simulink model "Scenario_MinimumExample_TwithoutTrafficLights_tol"  (R2021a)
settings: Solver=VariableStepAuto  StartTime=0.0  StopTime=50  RelTol=1e-3
model workspace (MAT data in the model file):
  Kz_dif = Simulink.Parameter
  Kz_dif.Value = Simulink.data.Expression
  Kz_dif.Value.ExpressionString = " L_dif / (Lc + ds)"
  Kz_dif.DataType = 'auto'
  Kz_dif.Dimensions = -1
  Kz_il = Simulink.Parameter
  Kz_il.Value = Simulink.data.Expression
  Kz_il.Value.ExpressionString = " L_il / (Lc + ds)"
  Kz_il.DataType = 'auto'
  Kz_il.Dimensions = -1
  Kz_ir = Simulink.Parameter
  Kz_ir.Value = Simulink.data.Expression
  Kz_ir.Value.ExpressionString = " L_ir / (Lc + ds)"
  Kz_ir.DataType = 'auto'
  Kz_ir.Dimensions = -1
  Kz_is = Simulink.Parameter
  Kz_is.Value = Simulink.data.Expression
  Kz_is.Value.ExpressionString = " L_is / (Lc + ds)"
  Kz_is.DataType = 'auto'
  Kz_is.Dimensions = -1
  Kz_long = Simulink.Parameter
  Kz_long.Value = Simulink.data.Expression
  Kz_long.Value.ExpressionString = " L_long / (Lc + ds)"
  Kz_long.Description = 'Segmentkapazität (wie viele autos passen hinein)'
  Kz_long.DataType = 'auto'
  Kz_long.Dimensions = -1
  Kz_pre = Simulink.Parameter
  Kz_pre.Value = Simulink.data.Expression
  Kz_pre.Value.ExpressionString = " L_pre / (Lc + ds)"
  Kz_pre.DataType = 'auto'
  Kz_pre.Dimensions = -1
  L_dif = Simulink.Parameter
  L_dif.Value = Simulink.data.Expression
  L_dif.Value.ExpressionString = "L_long-L_pre"
  L_dif.Description = 'Differenz zwischen Abbiegerspurlänge und normaler straßenlänge'
  L_dif.DataType = 'auto'
  L_dif.Dimensions = -1
  L_il = Simulink.Parameter
  L_il.Value = 30
  L_il.Description = 'Länge der innenkreuzungssegments, das linksabbieger durchqueren'
  L_il.DataType = 'auto'
  L_il.Dimensions = [1 1]
  L_ir = Simulink.Parameter
  L_ir.Value = 23
  L_ir.Description = 'Länge der innenkreuzungssegments, das rechtsabbieger durchqueren'
  L_ir.DataType = 'auto'
  L_ir.Dimensions = [1 1]
  L_is = Simulink.Parameter
  L_is.Value = 35
  L_is.Description = 'Länge der innenkreuzungssegments, das geradeausfahrer durchqueren'
  L_is.DataType = 'auto'
  L_is.Dimensions = [1 1]
  L_long = Simulink.Parameter
  L_long.Value = 52.8
  L_long.Description = 'Langes straßensegment  (52.8 meter)'
  L_long.DataType = 'auto'
  L_long.Dimensions = [1 1]
  L_pre = Simulink.Parameter
  L_pre.Value = 20
  L_pre.Description = 'Länge der Abbiegespuren'
  L_pre.DataType = 'auto'
  L_pre.Dimensions = [1 1]
  Lc = Simulink.Parameter
  Lc.Value = 4.4
  Lc.Description = 'Länge eines autos'
  Lc.DataType = 'auto'
  Lc.Dimensions = [1 1]
  Rk = Simulink.Parameter
  Rk.Value = Simulink.data.Expression
  Rk.Value.ExpressionString = " 1 / (Lc / v)"
  Rk.Description = 'Flussrate zwischen den Kanten (bei speed v)'
  Rk.DataType = 'auto'
  Rk.Dimensions = -1
  Tz_dif = Simulink.Parameter
  Tz_dif.Value = Simulink.data.Expression
  Tz_dif.Value.ExpressionString = " L_dif / v"
  Tz_dif.DataType = 'auto'
  Tz_dif.Dimensions = -1
  Tz_il = Simulink.Parameter
  Tz_il.Value = Simulink.data.Expression
  Tz_il.Value.ExpressionString = " L_il / v"
  Tz_il.DataType = 'auto'
  Tz_il.Dimensions = -1
  Tz_ir = Simulink.Parameter
  Tz_ir.Value = Simulink.data.Expression
  Tz_ir.Value.ExpressionString = " L_ir / v"
  Tz_ir.DataType = 'auto'
  Tz_ir.Dimensions = -1
  Tz_is = Simulink.Parameter
  Tz_is.Value = Simulink.data.Expression
  Tz_is.Value.ExpressionString = " L_is / v"
  Tz_is.DataType = 'auto'
  Tz_is.Dimensions = -1
  Tz_long = Simulink.Parameter
  Tz_long.Value = Simulink.data.Expression
  Tz_long.Value.ExpressionString = " L_long / v"
  Tz_long.Description = 'Segment durchfahrtzeit: wie lange würde ein auto brauchen,um
    | ungehindert durch das segment zu fahren.'
  Tz_long.DataType = 'auto'
  Tz_long.Dimensions = -1
  Tz_pre = Simulink.Parameter
  Tz_pre.Value = Simulink.data.Expression
  Tz_pre.Value.ExpressionString = " L_pre / v"
  Tz_pre.DataType = 'auto'
  Tz_pre.Dimensions = -1
  ds = Simulink.Parameter
  ds.Value = Simulink.data.Expression
  ds.Value.ExpressionString = "v*dt"
  ds.DataType = 'auto'
  ds.Dimensions = -1
  dt = Simulink.Parameter
  dt.Value = 1
  dt.Description = 'temporaler sicherheitsabstand'
  dt.DataType = 'auto'
  dt.Dimensions = [1 1]
  v = Simulink.Parameter
  v.Value = 13.89
  v.Description = 'geschwindigkeit eines autos
    | (km/h : 3.75 = m/s)
    | 	30km/h = 8,34m/s
    | 	20km/h = 5.56m/s
    | 	50km/h = 13.89m/s
    | '
  v.DataType = 'auto'
  v.Dimensions = [1 1]
libraries: StreetLanesLibrary x72, EdgesLibrary x64, MeasuringLibrary x34, SourcesAndSinksLibrary x11
(part 1 of 2)
settings Model: Creator=phill  LastModifiedBy=phill
settings SolverCC: ZeroCrossAlgorithm=Adaptive

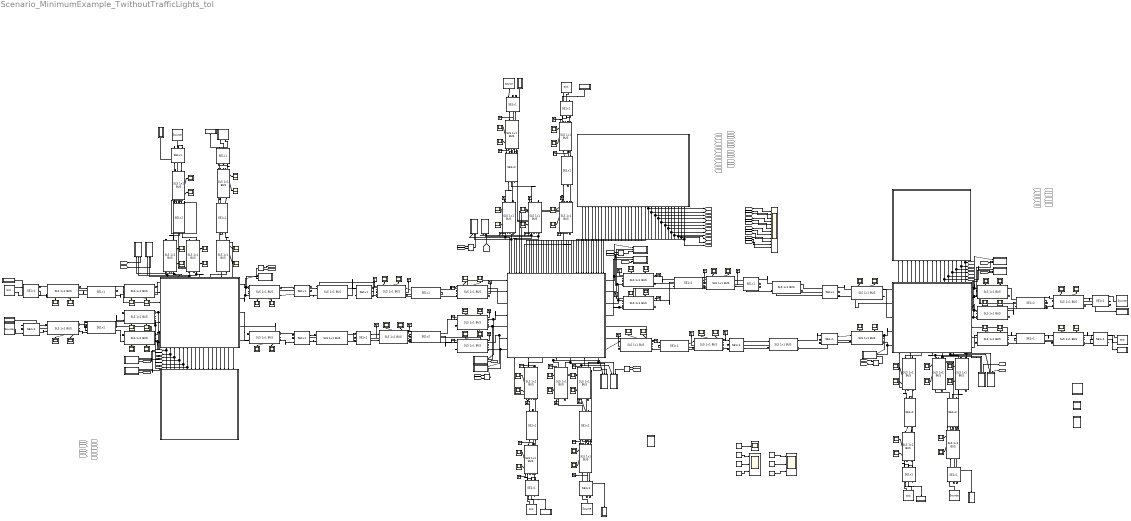
== system Scenario_MinimumExample_TwithoutTrafficLights_tol ==
  note: Controllers with tolerance
  Ain : StreetLanesLibrary/SLS 1x1 BUS  Kz=Kz_dif  Tz=Tz_dif
  Ain1 : StreetLanesLibrary/SLS 1x1 BUS  Kz=Kz_dif  Tz=Tz_dif
  Ain2 : StreetLanesLibrary/SLS 1x1 BUS  Kz=Kz_dif  Tz=Tz_dif
  AinSplit : EdgesLibrary/SE1x2  Rk1=0.5*Rk  Rk2=0.5*Rk
  AinSplit1 : EdgesLibrary/SE1x2  Rk1=0.5*Rk  Rk2=0.5*Rk
  AinSplit2 : EdgesLibrary/SE1x2  Rk1=0.5*Rk  Rk2=0.5*Rk
  AinX : Scope
  AinX1 : Scope
  AinX2 : Scope
  AinY : Scope
  AinY1 : Scope
  AinY2 : Scope
  Al : StreetLanesLibrary/SLS 1x1 BUS  Kz=Kz_pre  Tz=Tz_pre
  AlX : Scope
  AlY : Scope
  Ali : StreetLanesLibrary/SLS 1x1 BUS  Kz=Kz_pre  Tz=Tz_pre
  Ali1 : StreetLanesLibrary/SLS 1x1 BUS  Kz=Kz_pre  Tz=Tz_pre
  AliX : Scope
  AliX1 : Scope
  AliY : Scope
  AliY1 : Scope
  Ao : StreetLanesLibrary/SLS 1x1 BUS  Kz=Kz_pre  Tz=Tz_pre
  Ao1 : StreetLanesLibrary/SLS 1x1 BUS  Kz=Kz_pre  Tz=Tz_pre
  Ao2 : StreetLanesLibrary/SLS 1x1 BUS  Kz=Kz_pre  Tz=Tz_pre
  AoX : Scope
  AoX1 : Scope
  AoX2 : Scope
  AoY : Scope
  AoY1 : Scope
  AoY2 : Scope
  Aout : StreetLanesLibrary/SLS 1x1 BUS  Kz=Kz_dif  Tz=Tz_dif
  Aout1 : StreetLanesLibrary/SLS 1x1 BUS  Kz=Kz_dif  Tz=Tz_dif
  Aout2 : StreetLanesLibrary/SLS 1x1 BUS  Kz=Kz_dif  Tz=Tz_dif
  AoutX : Scope
  AoutX1 : Scope
  AoutX2 : Scope
  AoutY : Scope
  AoutY1 : Scope
  AoutY2 : Scope
  Ari : StreetLanesLibrary/SLS 1x1 BUS  Kz=Kz_pre  Tz=Tz_pre
  Ari1 : StreetLanesLibrary/SLS 1x1 BUS  Kz=Kz_pre  Tz=Tz_pre
  AriX : Scope
  AriX1 : Scope
  AriY : Scope
  AriY1 : Scope
  Ars : StreetLanesLibrary/SLS 1x1 BUS  Kz=Kz_pre  Tz=Tz_pre
  ArsX : Scope
  ArsY : Scope
  Bin : StreetLanesLibrary/SLS 1x1 BUS  Kz=Kz_dif  Tz=Tz_dif
  BinSplit1 : EdgesLibrary/SE1x2  Rk1=0.5*Rk  Rk2=0.5*Rk
  BinX : Scope
  BinY : Scope
  Bl : StreetLanesLibrary/SLS 1x1 BUS  Kz=Kz_pre  Tz=Tz_pre
  BlX : Scope
  BlY : Scope
  Bo : StreetLanesLibrary/SLS 1x1 BUS  Kz=Kz_pre  Tz=Tz_pre
  Bo1 : StreetLanesLibrary/SLS 1x1 BUS  Kz=Kz_pre  Tz=Tz_pre
  Bo2 : StreetLanesLibrary/SLS 1x1 BUS  Kz=Kz_pre  Tz=Tz_pre
  Bo3 : StreetLanesLibrary/SLS 1x1 BUS  Kz=Kz_long  Tz=Tz_long
  BoX : Scope
  BoX1 : Scope
  BoX2 : Scope
  BoY : Scope
  BoY1 : Scope
  BoY2 : Scope
  Bout : StreetLanesLibrary/SLS 1x1 BUS  Kz=Kz_dif  Tz=Tz_dif
  BoutX : Scope
  BoutY : Scope
  Brs : StreetLanesLibrary/SLS 1x1 BUS  Kz=Kz_pre  Tz=Tz_pre
  Brs1 : StreetLanesLibrary/SLS 1x1 BUS  Kz=Kz_pre  Tz=Tz_pre
  Brs2 : StreetLanesLibrary/SLS 1x1 BUS  Kz=Kz_pre  Tz=Tz_pre
  Brs3 : StreetLanesLibrary/SLS 1x1 BUS  Kz=Kz_long  Tz=Tz_long
  BrsX : Scope
  BrsX1 : Scope
  BrsX2 : Scope
  BrsY : Scope
  BrsY1 : Scope
  BrsY2 : Scope
  Chart1 : Stateflow chart  TreatAsAtomicUnit=on  mask{tol=0}
      mask prompts: tol "tolerance"
      settings: PortSchema="{\"entries\":[{\"content\":{\"sides\":[{\"content\":{\"connectorIds\":[]},\"type\":\"ConnectorPlacement.EquallySpacedRectSide\",\"uuid\":\"dee1a780-e9dd-4205-adb9-3e9cb1ec0cd6\"},{\"content\":{\"connectorIds\":[],\"side\":\"RIGHT\"},\"type\":\"ConnectorPlacement.EquallySpacedRectSide\",\"uuid\":\"bc6af08d-2df8-4a74-93d0-032b7c1c381c\"},{\"content\":{\"connectorIds\":[],\"side\":\"TOP\"},\"type\":\"ConnectorPlacement.EquallySpacedRectSide\",\"uuid\":\"98fea325-c9fc-472d-8e1a-d846d6e99e12\"},{\"content\":{\"connectorIds\":[\"In5\",\"In1\",\"In2\",\"In3\",\"In4\",\"In11\",\"In10\",\"In9\",\"In8\",\"In7\",\"In6\",\"Out5\",\"Out6\",\"Out1\",\"Out2\",\"Out3\",\"Out4\"],\"side\":\"BOTTOM\"},\"type\":\"ConnectorPlacement.EquallySpacedRectSide\",\"uuid\":\"a092283f-ef46-48e2-a5f8-8210ac00b2f9\"}]},\"type\":\"ConnectorPlacement.EquallySpacedConnector\",\"uuid\":\"33a851aa-4180-41c0-b4bb-9b9c3be41936\"}],\"packageUris\":[\"http://schema.mathworks.com/mf0/Connector/R2020b\"],\"version\":\"1.0\"}"
  Chart2 : Stateflow chart  TreatAsAtomicUnit=on  mask{tol=0}
      mask prompts: tol "tolerance"
      settings: PortSchema="{\"entries\":[{\"content\":{\"sides\":[{\"content\":{\"connectorIds\":[]},\"type\":\"ConnectorPlacement.EquallySpacedRectSide\",\"uuid\":\"dee1a780-e9dd-4205-adb9-3e9cb1ec0cd6\"},{\"content\":{\"connectorIds\":[],\"side\":\"RIGHT\"},\"type\":\"ConnectorPlacement.EquallySpacedRectSide\",\"uuid\":\"bc6af08d-2df8-4a74-93d0-032b7c1c381c\"},{\"content\":{\"connectorIds\":[],\"side\":\"TOP\"},\"type\":\"ConnectorPlacement.EquallySpacedRectSide\",\"uuid\":\"98fea325-c9fc-472d-8e1a-d846d6e99e12\"},{\"content\":{\"connectorIds\":[\"In5\",\"In1\",\"In2\",\"In3\",\"In4\",\"In11\",\"In10\",\"In9\",\"In8\",\"In7\",\"In6\",\"Out5\",\"Out6\",\"Out1\",\"Out2\",\"Out3\",\"Out4\"],\"side\":\"BOTTOM\"},\"type\":\"ConnectorPlacement.EquallySpacedRectSide\",\"uuid\":\"a092283f-ef46-48e2-a5f8-8210ac00b2f9\"}]},\"type\":\"ConnectorPlacement.EquallySpacedConnector\",\"uuid\":\"33a851aa-4180-41c0-b4bb-9b9c3be41936\"}],\"packageUris\":[\"http://schema.mathworks.com/mf0/Connector/R2020b\"],\"version\":\"1.0\"}"
  Cin : StreetLanesLibrary/SLS 1x1 BUS  Kz=Kz_dif  Tz=Tz_dif
  Cin1 : StreetLanesLibrary/SLS 1x1 BUS  Kz=Kz_dif  Tz=Tz_dif
  Cin2 : StreetLanesLibrary/SLS 1x1 BUS  Kz=Kz_dif  Tz=Tz_dif
  Cin3 : StreetLanesLibrary/SLS 1x1 BUS  Kz=Kz_long  Tz=Tz_long
  CinSplit : EdgesLibrary/SE1x2  Rk1=0.5*Rk  Rk2=0.5*Rk
  CinSplit1 : EdgesLibrary/SE1x2  Rk1=0.5*Rk  Rk2=0.5*Rk
  CinSplit2 : EdgesLibrary/SE1x2  Rk1=0.5*Rk  Rk2=0.5*Rk
  CinX : Scope
  CinX1 : Scope
  CinX2 : Scope
  CinY : Scope
  CinY1 : Scope
  CinY2 : Scope
  Cl : StreetLanesLibrary/SLS 1x1 BUS  Kz=Kz_pre  Tz=Tz_pre
  Cl1 : StreetLanesLibrary/SLS 1x1 BUS  Kz=Kz_pre  Tz=Tz_pre
  Cl2 : StreetLanesLibrary/SLS 1x1 BUS  Kz=Kz_pre  Tz=Tz_pre
  ClX : Scope
  ClX1 : Scope
  ClX2 : Scope
  ClY : Scope
  ClY1 : Scope
  Cly : Scope
  Co : StreetLanesLibrary/SLS 1x1 BUS  Kz=Kz_pre  Tz=Tz_pre
  Co1 : StreetLanesLibrary/SLS 1x1 BUS  Kz=Kz_pre  Tz=Tz_pre
  Co2 : StreetLanesLibrary/SLS 1x1 BUS  Kz=Kz_pre  Tz=Tz_pre
  CoX : Scope
  CoX1 : Scope
  CoX2 : Scope
  CoY : Scope
  CoY1 : Scope
  CoY2 : Scope
  Cout{,1..3} (4 alike) : StreetLanesLibrary/SLS 1x1 BUS  Kz=Kz_dif  Tz=Tz_dif
  CoutX : Scope
  CoutX1 : Scope
  CoutX2 : Scope
  CoutY : Scope
  CoutY1 : Scope
  CoutY2 : Scope
  Crs : StreetLanesLibrary/SLS 1x1 BUS  Kz=Kz_pre  Tz=Tz_pre
  CrsX : Scope
  CrsY : Scope
  Cs : StreetLanesLibrary/SLS 1x1 BUS  Kz=Kz_pre  Tz=Tz_pre
  Cs1 : StreetLanesLibrary/SLS 1x1 BUS  Kz=Kz_pre  Tz=Tz_pre
  CsX : Scope
  CsX1 : Scope
  CsY : Scope
  CsY1 : Scope
  Din : StreetLanesLibrary/SLS 1x1 BUS  Kz=Kz_dif  Tz=Tz_dif
  DinSplit : EdgesLibrary/SE1x2  Rk1=0.5*Rk  Rk2=0.5*Rk
  DinX : Scope
  DinY : Scope
  Dl : StreetLanesLibrary/SLS 1x1 BUS  Kz=Kz_pre  Tz=Tz_pre
  DlX : Scope
  DlY : Scope
  Do : StreetLanesLibrary/SLS 1x1 BUS  Kz=Kz_pre  Tz=Tz_pre
  DoX : Scope
  DoY : Scope
  Dout : StreetLanesLibrary/SLS 1x1 BUS  Kz=Kz_dif  Tz=Tz_dif
  DoutX : Scope
  DoutY : Scope
  Drs : StreetLanesLibrary/SLS 1x1 BUS  Kz=Kz_pre  Tz=Tz_pre
  DrsX : Scope
  DrsY : Scope
  From14 : From  Commented=on  GotoTag=LenCs
  From15 : From  Commented=on  GotoTag=LenCl
  From20 : From  Commented=on  GotoTag=LenAr
  From21 : From  Commented=on  GotoTag=LenAl
  From22 : From  Commented=on  GotoTag=LenBr
  From23 : From  Commented=on  GotoTag=LenBs
  From24 : From  Commented=on  GotoTag=CenAl
  From25 : From  Commented=on  GotoTag=CenAs
  From26 : From  Commented=on  GotoTag=CenDs
  From27 : From  Commented=on  GotoTag=CenDr
  From28 : From  Commented=on  GotoTag=CenAr
  From29 : From  Commented=on  GotoTag=CenBl
  From30 : From  Commented=on  GotoTag=CenBs
  From31 : From  Commented=on  GotoTag=CenBr
  From32 : From  Commented=on  GotoTag=CenCl
  From33 : From  Commented=on  GotoTag=CenCs
  From34 : From  Commented=on  GotoTag=CenCr
  From35 : From  Commented=on  GotoTag=CenDl
  From42 : From  Commented=on  GotoTag=RenCs
  From43 : From  Commented=on  GotoTag=RenCl
  From44 : From  Commented=on  GotoTag=RenAr
  From45 : From  Commented=on  GotoTag=RenAl
  From46 : From  Commented=on  GotoTag=RenBr
  From47 : From  Commented=on  GotoTag=RenBs
  Goto12 : Goto  Commented=on  GotoTag=LenCl
  Goto13 : Goto  Commented=on  GotoTag=LenCs
  Goto16 : Goto  Commented=on  GotoTag=LenBs
  Goto17 : Goto  Commented=on  GotoTag=LenBr
  Goto18 : Goto  Commented=on  GotoTag=LenAl
  Goto19 : Goto  Commented=on  GotoTag=LenAr
  Goto24 : Goto  Commented=on  GotoTag=CenAl
  Goto25 : Goto  Commented=on  GotoTag=CenAs
  Goto26 : Goto  Commented=on  GotoTag=CenDs
  Goto27 : Goto  Commented=on  GotoTag=CenDr
  Goto28 : Goto  Commented=on  GotoTag=CenAr
  Goto29 : Goto  Commented=on  GotoTag=CenBl
  Goto30 : Goto  Commented=on  GotoTag=CenBs
  Goto31 : Goto  Commented=on  GotoTag=CenBr
  Goto32 : Goto  Commented=on  GotoTag=CenCl
  Goto33 : Goto  Commented=on  GotoTag=CenCs
  Goto34 : Goto  Commented=on  GotoTag=CenCr
  Goto35 : Goto  Commented=on  GotoTag=CenDl
  Goto42 : Goto  Commented=on  GotoTag=RenCl
  Goto43 : Goto  Commented=on  GotoTag=RenCs
  Goto44 : Goto  Commented=on  GotoTag=RenBs
  Goto45 : Goto  Commented=on  GotoTag=RenBr
  Goto46 : Goto  Commented=on  GotoTag=RenAl
  Goto47 : Goto  Commented=on  GotoTag=RenAr
  Kz_dif : Constant  Value=Kz_dif
  Kz_long : Constant  Value=Kz_long
  Kz_pre : Constant  Value=Kz_pre
  Kzs : Scope  NumInputPorts=3
  Logical Operator{,1..5} (6 alike) : Logic  Operator=OR  AllPortsSameDT=off  OutDataTypeStr=boolean
  Plus-Controller : Stateflow chart  TreatAsAtomicUnit=on  mask{green_duration_sr=6, green_duration_l=6, tol=0}
      mask prompts: green_duration_sr "Green Duration for straight/right traffic"; green_duration_l "Green Duration for left traffic"; tol "tolerance"
      settings: PortSchema="{\"entries\":[{\"content\":{\"sides\":[{\"content\":{\"connectorIds\":[]},\"type\":\"ConnectorPlacement.EquallySpacedRectSide\",\"uuid\":\"2590cc03-86a2-4387-8b1b-fdf4c8b68aa6\"},{\"content\":{\"connectorIds\":[],\"side\":\"RIGHT\"},\"type\":\"ConnectorPlacement.EquallySpacedRectSide\",\"uuid\":\"b97063cd-dd31-425f-b4aa-3aaa013ac411\"},{\"content\":{\"connectorIds\":[],\"side\":\"TOP\"},\"type\":\"ConnectorPlacement.EquallySpacedRectSide\",\"uuid\":\"ef5846b9-436e-4b10-a854-1305521b6a0d\"},{\"content\":{\"connectorIds\":[\"In3\",\"In4\",\"In1\",\"In2\",\"In5\",\"In6\",\"In7\",\"In8\",\"In9\",\"In10\",\"In11\",\"In12\",\"In13\",\"In14\",\"In15\",\"In16\",\"In17\",\"In18\",\"In19\",\"In20\",\"Out1\",\"Out2\",\"Out3\",\"Out4\",\"Out5\",\"Out6\",\"Out7\",\"Out8\",\"Out9\",\"Out10\",\"Out11\",\"Out12\"],\"side\":\"BOTTOM\"},\"type\":\"ConnectorPlacement.EquallySpacedRectSide\",\"uuid\":\"44b73820-3b7c-4ee5-b5da-9465e85a924e\"}]},\"type\":\"ConnectorPlacement.EquallySpacedConnector\",\"uuid\":\"3342797d-7762-4a2a-891a-654024402a66\"}],\"packageUris\":[\"http://schema.mathworks.com/mf0/Connector/R2020b\"],\"version\":\"1.0\"}"
  Rk : Constant  Value=Rk
  SE1x{1..8} (8 alike) : EdgesLibrary/SE1x1  Rk=Rk  slope=2000
  Scope : Scope  NumInputPorts=12
  Sink A : SourcesAndSinksLibrary/Sink  SystemSampleTime=-1  VariantActivationTime=update diagram  Latency=0  AutoFrameSizeCalculation=off
      settings: PortSchema="{\"entries\":[{\"content\":{\"sides\":[{\"content\":{\"connectorIds\":[\"Out1\",\"Out2\"]},\"type\":\"ConnectorPlacement.EquallySpacedRectSide\",\"uuid\":\"9fd2383e-3590-4f0f-bafc-5a4adfbb32b4\"},{\"content\":{\"connectorIds\":[],\"side\":\"RIGHT\"},\"type\":\"ConnectorPlacement.EquallySpacedRectSide\",\"uuid\":\"1e687aa9-1098-45bd-a1f6-ea403f3f2897\"},{\"content\":{\"connectorIds\":[],\"side\":\"TOP\"},\"type\":\"ConnectorPlacement.EquallySpacedRectSide\",\"uuid\":\"fe6eaa71-085c-414b-983a-a0e72e52a49c\"}]},\"type\":\"ConnectorPlacement.EquallySpacedConnector\",\"uuid\":\"370c1712-4373-4726-99c2-6cb04807ece1\"}],\"packageUris\":[\"http://schema.mathworks.com/mf0/Connector/R2020b\"],\"version\":\"1.0\"}"
  Sink A1 : SourcesAndSinksLibrary/Sink  SystemSampleTime=-1  VariantActivationTime=update diagram  Latency=0  AutoFrameSizeCalculation=off
      settings: PortSchema="{\"entries\":[{\"content\":{\"sides\":[{\"content\":{\"connectorIds\":[\"Out1\",\"Out2\"]},\"type\":\"ConnectorPlacement.EquallySpacedRectSide\",\"uuid\":\"9fd2383e-3590-4f0f-bafc-5a4adfbb32b4\"},{\"content\":{\"connectorIds\":[],\"side\":\"RIGHT\"},\"type\":\"ConnectorPlacement.EquallySpacedRectSide\",\"uuid\":\"1e687aa9-1098-45bd-a1f6-ea403f3f2897\"},{\"content\":{\"connectorIds\":[],\"side\":\"TOP\"},\"type\":\"ConnectorPlacement.EquallySpacedRectSide\",\"uuid\":\"fe6eaa71-085c-414b-983a-a0e72e52a49c\"}]},\"type\":\"ConnectorPlacement.EquallySpacedConnector\",\"uuid\":\"370c1712-4373-4726-99c2-6cb04807ece1\"}],\"packageUris\":[\"http://schema.mathworks.com/mf0/Connector/R2020b\"],\"version\":\"1.0\"}"
  Sink A2 : Subsystem  AncestorBlock=SourcesAndSinksLibrary/Sink
      settings: PortSchema="{\"entries\":[{\"content\":{\"sides\":[{\"content\":{\"connectorIds\":[\"Out1\",\"Out2\"]},\"type\":\"ConnectorPlacement.EquallySpacedRectSide\",\"uuid\":\"9fd2383e-3590-4f0f-bafc-5a4adfbb32b4\"},{\"content\":{\"connectorIds\":[],\"side\":\"RIGHT\"},\"type\":\"ConnectorPlacement.EquallySpacedRectSide\",\"uuid\":\"1e687aa9-1098-45bd-a1f6-ea403f3f2897\"},{\"content\":{\"connectorIds\":[],\"side\":\"TOP\"},\"type\":\"ConnectorPlacement.EquallySpacedRectSide\",\"uuid\":\"fe6eaa71-085c-414b-983a-a0e72e52a49c\"}]},\"type\":\"ConnectorPlacement.EquallySpacedConnector\",\"uuid\":\"370c1712-4373-4726-99c2-6cb04807ece1\"}],\"packageUris\":[\"http://schema.mathworks.com/mf0/Connector/R2020b\"],\"version\":\"1.0\"}"
      mask Display: image('$imagefile'); % Use "Edit Image" on toolstrip to change.
  Sink C1 : SourcesAndSinksLibrary/Sink  SystemSampleTime=-1  VariantActivationTime=update diagram  Latency=0  AutoFrameSizeCalculation=off
      settings: PortSchema="{\"entries\":[{\"content\":{\"sides\":[{\"content\":{\"connectorIds\":[\"Out1\",\"Out2\"]},\"type\":\"ConnectorPlacement.EquallySpacedRectSide\",\"uuid\":\"9fd2383e-3590-4f0f-bafc-5a4adfbb32b4\"},{\"content\":{\"connectorIds\":[],\"side\":\"RIGHT\"},\"type\":\"ConnectorPlacement.EquallySpacedRectSide\",\"uuid\":\"1e687aa9-1098-45bd-a1f6-ea403f3f2897\"},{\"content\":{\"connectorIds\":[],\"side\":\"TOP\"},\"type\":\"ConnectorPlacement.EquallySpacedRectSide\",\"uuid\":\"fe6eaa71-085c-414b-983a-a0e72e52a49c\"}]},\"type\":\"ConnectorPlacement.EquallySpacedConnector\",\"uuid\":\"370c1712-4373-4726-99c2-6cb04807ece1\"}],\"packageUris\":[\"http://schema.mathworks.com/mf0/Connector/R2020b\"],\"version\":\"1.0\"}"
  Sink C2 : SourcesAndSinksLibrary/Sink  SystemSampleTime=-1  VariantActivationTime=update diagram  Latency=0  AutoFrameSizeCalculation=off
      settings: PortSchema="{\"entries\":[{\"content\":{\"sides\":[{\"content\":{\"connectorIds\":[\"Out1\",\"Out2\"]},\"type\":\"ConnectorPlacement.EquallySpacedRectSide\",\"uuid\":\"9fd2383e-3590-4f0f-bafc-5a4adfbb32b4\"},{\"content\":{\"connectorIds\":[],\"side\":\"RIGHT\"},\"type\":\"ConnectorPlacement.EquallySpacedRectSide\",\"uuid\":\"1e687aa9-1098-45bd-a1f6-ea403f3f2897\"},{\"content\":{\"connectorIds\":[],\"side\":\"TOP\"},\"type\":\"ConnectorPlacement.EquallySpacedRectSide\",\"uuid\":\"fe6eaa71-085c-414b-983a-a0e72e52a49c\"}]},\"type\":\"ConnectorPlacement.EquallySpacedConnector\",\"uuid\":\"370c1712-4373-4726-99c2-6cb04807ece1\"}],\"packageUris\":[\"http://schema.mathworks.com/mf0/Connector/R2020b\"],\"version\":\"1.0\"}"
  Sink D : SourcesAndSinksLibrary/Sink  SystemSampleTime=-1  VariantActivationTime=update diagram  Latency=0  AutoFrameSizeCalculation=off
      settings: PortSchema="{\"entries\":[{\"content\":{\"sides\":[{\"content\":{\"connectorIds\":[\"Out1\",\"Out2\"]},\"type\":\"ConnectorPlacement.EquallySpacedRectSide\",\"uuid\":\"9fd2383e-3590-4f0f-bafc-5a4adfbb32b4\"},{\"content\":{\"connectorIds\":[],\"side\":\"RIGHT\"},\"type\":\"ConnectorPlacement.EquallySpacedRectSide\",\"uuid\":\"1e687aa9-1098-45bd-a1f6-ea403f3f2897\"},{\"content\":{\"connectorIds\":[],\"side\":\"TOP\"},\"type\":\"ConnectorPlacement.EquallySpacedRectSide\",\"uuid\":\"fe6eaa71-085c-414b-983a-a0e72e52a49c\"}]},\"type\":\"ConnectorPlacement.EquallySpacedConnector\",\"uuid\":\"370c1712-4373-4726-99c2-6cb04807ece1\"}],\"packageUris\":[\"http://schema.mathworks.com/mf0/Connector/R2020b\"],\"version\":\"1.0\"}"
  Source A : SourcesAndSinksLibrary/Source  SystemSampleTime=-1  VariantActivationTime=update diagram  Latency=0  AutoFrameSizeCalculation=off
  Source A1 : SourcesAndSinksLibrary/Source  SystemSampleTime=-1  VariantActivationTime=update diagram  Latency=0  AutoFrameSizeCalculation=off
  Source A2 : SourcesAndSinksLibrary/Source  SystemSampleTime=-1  VariantActivationTime=update diagram  Latency=0  AutoFrameSizeCalculation=off
  Source C1 : SourcesAndSinksLibrary/Source  SystemSampleTime=-1  VariantActivationTime=update diagram  Latency=0  AutoFrameSizeCalculation=off
  Source C2 : SourcesAndSinksLibrary/Source  SystemSampleTime=-1  VariantActivationTime=update diagram  Latency=0  AutoFrameSizeCalculation=off
  Source D : SourcesAndSinksLibrary/Source  SystemSampleTime=-1  VariantActivationTime=update diagram  Latency=0  AutoFrameSizeCalculation=off
  Subsystem : Subsystem  mask{Kz_left=Kz_il, Tz_left=Tz_il, Kz_straight=Kz_is, Tz_straight=Tz_is, Kz_right=Kz_ir, Tz_right=Tz_ir, Rk=Rk}
      settings: PortSchema="{\"entries\":[{\"content\":{\"sides\":[{\"content\":{\"connectorIds\":[\"In1\",\"In2\",\"Out30\",\"In3\",\"Out31\",\"In4\",\"Out32\"]},\"type\":\"ConnectorPlacement.EquallySpacedRectSide\",\"uuid\":\"223afcc5-5490-41e2-b2c1-0ac31bdd31f0\"},{\"content\":{\"connectorIds\":[\"In25\",\"Out1\",\"In26\",\"Out2\",\"In27\",\"In28\",\"Out3\"],\"side\":\"RIGHT\"},\"type\":\"ConnectorPlacement.EquallySpacedRectSide\",\"uuid\":\"e803e5ea-345a-49fc-8782-ffb100729ba0\"},{\"content\":{\"connectorIds\":[\"In5\",\"Out7\",\"Out8\",\"In6\",\"In7\",\"In8\",\"Out9\",\"Out10\",\"Out11\",\"Out12\",\"Out13\",\"Out14\",\"Out15\",\"Out16\",\"Out17\",\"Out18\",\"Out19\",\"Out20\",\"Out21\",\"Out22\",\"Out23\",\"Out24\",\"Out25\",\"Out26\",\"Out27\",\"Out28\",\"Out29\",\"In9\",\"In10\",\"In11\",\"In12\",\"In13\",\"In14\",\"In15\",\"In16\",\"In17\",\"In18\",\"In19\",\"In20\"],\"side\":\"TOP\"},\"type\":\"ConnectorPlacement.EquallySpacedRectSide\",\"uuid\":\"8581fbf9-6742-4a7a-9e93-ed29b1a56c31\"},{\"content\":{\"connectorIds\":[\"In21\",\"In22\",\"Out4\",\"In23\",\"Out5\",\"In24\",\"Out6\"],\"side\":\"BOTTOM\"},\"type\":\"ConnectorPlacement.EquallySpacedRectSide\",\"uuid\":\"cc67de78-9dd9-463d-9445-caa2eb7c099b\"}]},\"type\":\"ConnectorPlacement.EquallySpacedConnector\",\"uuid\":\"ac6fc4cc-2326-4bcf-896c-a5d089a8f47a\"}],\"packageUris\":[\"http://schema.mathworks.com/mf0/Connector/R2020b\"],\"version\":\"1.0\"}"
      mask Display:
      | %image('$imagefile'); % Use "Edit Image" on toolstrip to change.
      | disp('+ \n\n');
      | KzS = get_param(gcb,'Kz_straight');
      | TzS = get_param(gcb,'Tz_straight');
      | KzR = get_param(gcb,'Kz_right');
      | TzR = get_param(gcb,'Tz_right');
      | KzL = get_param(gcb,'Kz_left');
      | TzL = get_param(gcb,'Tz_left');
      | Rk = get_param(gcb,'Rk');
      | disp(['Rk = ', Rk, ' | Kz/Tz L = ', KzL, ' ', TzL, ' | Kz/Tz S = ', KzS, ' ', TzS, ' | Kz/Tz R = ', KzR, ' ', TzR]);
  Subsystem1 : Subsystem  mask{Kz_left=Kz_il, Tz_left=Tz_il, Kz_straight=Kz_is, Tz_straight=Tz_is, Kz_right=Kz_ir, Tz_right=Tz_ir, Rk=Rk}
      settings: PortSchema="{\"entries\":[{\"content\":{\"sides\":[{\"content\":{\"connectorIds\":[\"In1\",\"In2\",\"Out18\",\"In3\",\"Out19\"]},\"type\":\"ConnectorPlacement.EquallySpacedRectSide\",\"uuid\":\"96c9f498-b0bc-4839-a476-8992d885d35a\"},{\"content\":{\"connectorIds\":[\"In14\",\"Out1\",\"In15\",\"Out2\",\"In16\",\"In17\",\"Out3\"],\"side\":\"RIGHT\"},\"type\":\"ConnectorPlacement.EquallySpacedRectSide\",\"uuid\":\"11ab0cdd-7db6-4f39-a252-8216aa6322d2\"},{\"content\":{\"connectorIds\":[\"Out7\",\"Out8\",\"Out9\",\"Out10\",\"Out11\",\"Out12\",\"Out13\",\"Out14\",\"Out15\",\"Out16\",\"Out17\",\"In4\",\"In5\",\"In6\",\"In7\",\"In8\",\"In9\"],\"side\":\"TOP\"},\"type\":\"ConnectorPlacement.EquallySpacedRectSide\",\"uuid\":\"f8ff7b80-df82-4633-b83a-80e44c4409b9\"},{\"content\":{\"connectorIds\":[\"In10\",\"In11\",\"Out4\",\"In12\",\"Out5\",\"In13\",\"Out6\"],\"side\":\"BOTTOM\"},\"type\":\"ConnectorPlacement.EquallySpacedRectSide\",\"uuid\":\"816219a6-152c-447e-807e-ad4d62c96b47\"}]},\"type\":\"ConnectorPlacement.EquallySpacedConnector\",\"uuid\":\"16c591aa-9a6b-4cb9-9c60-a78ca06e8a6b\"}],\"packageUris\":[\"http://schema.mathworks.com/mf0/Connector/R2020b\"],\"version\":\"1.0\"}"
      mask Display:
      | %image('$imagefile'); % Use "Edit Image" on toolstrip to change.
      | disp('T \n\n');
      | KzS = get_param(gcb,'Kz_straight');
      | TzS = get_param(gcb,'Tz_straight');
      | KzR = get_param(gcb,'Kz_right');
      | TzR = get_param(gcb,'Tz_right');
      | KzL = get_param(gcb,'Kz_left');
      | TzL = get_param(gcb,'Tz_left');
      | Rk = get_param(gcb,'Rk');
      | disp(['Rk = ', Rk, ' | Kz/Tz L = ', KzL, ' ', TzL, ' | Kz/Tz S = ', KzS, ' ', TzS, ' | Kz/Tz R = ', KzR, ' ', TzR]);
  Subsystem2 : Subsystem  mask{Kz_left=Kz_il, Tz_left=Tz_il, Kz_straight=Kz_is, Tz_straight=Tz_is, Kz_right=Kz_ir, Tz_right=Tz_ir, Rk=Rk}
      settings: PortSchema="{\"entries\":[{\"content\":{\"sides\":[{\"content\":{\"connectorIds\":[\"In1\",\"In2\",\"Out18\",\"In3\",\"Out19\"]},\"type\":\"ConnectorPlacement.EquallySpacedRectSide\",\"uuid\":\"96c9f498-b0bc-4839-a476-8992d885d35a\"},{\"content\":{\"connectorIds\":[\"In14\",\"Out1\",\"In15\",\"Out2\",\"In16\",\"In17\",\"Out3\"],\"side\":\"RIGHT\"},\"type\":\"ConnectorPlacement.EquallySpacedRectSide\",\"uuid\":\"11ab0cdd-7db6-4f39-a252-8216aa6322d2\"},{\"content\":{\"connectorIds\":[\"Out7\",\"Out8\",\"Out9\",\"Out10\",\"Out11\",\"Out12\",\"Out13\",\"Out14\",\"Out15\",\"Out16\",\"Out17\",\"In4\",\"In5\",\"In6\",\"In7\",\"In8\",\"In9\"],\"side\":\"TOP\"},\"type\":\"ConnectorPlacement.EquallySpacedRectSide\",\"uuid\":\"f8ff7b80-df82-4633-b83a-80e44c4409b9\"},{\"content\":{\"connectorIds\":[\"In10\",\"In11\",\"Out4\",\"In12\",\"Out5\",\"In13\",\"Out6\"],\"side\":\"BOTTOM\"},\"type\":\"ConnectorPlacement.EquallySpacedRectSide\",\"uuid\":\"816219a6-152c-447e-807e-ad4d62c96b47\"}]},\"type\":\"ConnectorPlacement.EquallySpacedConnector\",\"uuid\":\"16c591aa-9a6b-4cb9-9c60-a78ca06e8a6b\"}],\"packageUris\":[\"http://schema.mathworks.com/mf0/Connector/R2020b\"],\"version\":\"1.0\"}"
      mask Display:
      | %image('$imagefile'); % Use "Edit Image" on toolstrip to change.
      | disp('T \n\n');
      | KzS = get_param(gcb,'Kz_straight');
      | TzS = get_param(gcb,'Tz_straight');
      | KzR = get_param(gcb,'Kz_right');
      | TzR = get_param(gcb,'Tz_right');
      | KzL = get_param(gcb,'Kz_left');
      | TzL = get_param(gcb,'Tz_left');
      | Rk = get_param(gcb,'Rk');
      | disp(['Rk = ', Rk, ' | Kz/Tz L = ', KzL, ' ', TzL, ' | Kz/Tz S = ', KzS, ' ', TzS, ' | Kz/Tz R = ', KzR, ' ', TzR]);
  Terminator{1..7,10..16,19..25,28..34,37..48} (40 alike) : Terminator
  Tz_dif : Constant  Value=Tz_dif
  Tz_long : Constant  Value=Tz_long
  Tz_pre : Constant  Value=Tz_pre
  Tzs : Scope  NumInputPorts=3
  Tzs1 : Scope
  deadtimes : Subsystem  AncestorBlock=MeasuringLibrary/crossing_inflow_segment_checker_scope
  deadtimes1 : Subsystem  AncestorBlock=MeasuringLibrary/crossing_inflow_segment_checker_scope
  deadtimes10 : Subsystem  AncestorBlock=MeasuringLibrary/crossing_inflow_segment_checker_scope
  deadtimes11 : Subsystem  AncestorBlock=MeasuringLibrary/crossing_inflow_segment_checker_scope
  deadtimes12 : Subsystem  AncestorBlock=MeasuringLibrary/crossing_inflow_segment_checker_scope
  deadtimes13 : Subsystem  AncestorBlock=MeasuringLibrary/crossing_inflow_segment_checker_scope
  deadtimes14 : Subsystem  AncestorBlock=MeasuringLibrary/crossing_inflow_segment_checker_scope
  deadtimes15 : Subsystem  AncestorBlock=MeasuringLibrary/crossing_inflow_segment_checker_scope
  deadtimes16 : Subsystem  AncestorBlock=MeasuringLibrary/crossing_inflow_segment_checker_scope
  deadtimes17 : Subsystem  AncestorBlock=MeasuringLibrary/crossing_inflow_segment_checker_scope
  deadtimes2 : Subsystem  AncestorBlock=MeasuringLibrary/crossing_inflow_segment_checker_scope
  deadtimes3 : Subsystem  AncestorBlock=MeasuringLibrary/crossing_inflow_segment_checker_scope
  deadtimes4 : Subsystem  AncestorBlock=MeasuringLibrary/crossing_inflow_segment_checker_scope
  deadtimes5 : Subsystem  AncestorBlock=MeasuringLibrary/crossing_inflow_segment_checker_scope
  deadtimes6 : Subsystem  AncestorBlock=MeasuringLibrary/crossing_inflow_segment_checker_scope
  deadtimes7 : Subsystem  AncestorBlock=MeasuringLibrary/crossing_inflow_segment_checker_scope
  deadtimes8 : Subsystem  AncestorBlock=MeasuringLibrary/crossing_inflow_segment_checker_scope
  deadtimes9 : Subsystem  AncestorBlock=MeasuringLibrary/crossing_inflow_segment_checker_scope
  from Source A : EdgesLibrary/SE1x1  Rk=Rk  slope=2000
  from Source A1 : EdgesLibrary/SE1x1  Rk=Rk  slope=2000
  from Source A2 : EdgesLibrary/SE1x1  Rk=Rk  slope=2000
  from Source B : EdgesLibrary/SE1x1  Rk=Rk  slope=2000
  from Source B1 : EdgesLibrary/SE1x1  Rk=Rk  slope=2000
  from Source B2 : EdgesLibrary/SE1x1  Rk=Rk  slope=2000
  from Source C : EdgesLibrary/SE1x1  Rk=Rk  slope=2000
  from Source C1 : EdgesLibrary/SE1x1  Rk=Rk  slope=2000
  from Source C2 : EdgesLibrary/SE1x1  Rk=Rk  slope=2000
  from Source D : EdgesLibrary/SE1x1  Rk=Rk  slope=2000
  rel xz : Subsystem  AncestorBlock=MeasuringLibrary/rel xz scope
  sinks : Subsystem  AncestorBlock=MeasuringLibrary/sink_edge_checker_scope  mask{shortestPathTz=0}
      mask prompts: shortestPathTz "Sum of Tz on the path to the closest source"
      mask Display: disp(['pathTz = ', get_param(gcb,'shortestPathTz')])
  sinks1 : Subsystem  AncestorBlock=MeasuringLibrary/sink_edge_checker_scope  mask{shortestPathTz=2*Tz_dif+2*Tz_pre+Tz_ir}
      mask prompts: shortestPathTz "Sum of Tz on the path to the closest source"
      mask Display: disp(['pathTz = ', get_param(gcb,'shortestPathTz')])
  sinks2 : Subsystem  AncestorBlock=MeasuringLibrary/sink_edge_checker_scope  mask{shortestPathTz=2*Tz_dif+2*Tz_pre+Tz_il}
      mask prompts: shortestPathTz "Sum of Tz on the path to the closest source"
      mask Display: disp(['pathTz = ', get_param(gcb,'shortestPathTz')])
  sinks3 : Subsystem  AncestorBlock=MeasuringLibrary/sink_edge_checker_scope  mask{shortestPathTz=2*Tz_dif+2*Tz_pre+Tz_is}
      mask prompts: shortestPathTz "Sum of Tz on the path to the closest source"
      mask Display: disp(['pathTz = ', get_param(gcb,'shortestPathTz')])
  sinks4 : Subsystem  AncestorBlock=MeasuringLibrary/sink_edge_checker_scope  mask{shortestPathTz=2*Tz_dif+2*Tz_pre+Tz_is}
      mask prompts: shortestPathTz "Sum of Tz on the path to the closest source"
      mask Display: disp(['pathTz = ', get_param(gcb,'shortestPathTz')])
  sinks5 : Subsystem  AncestorBlock=MeasuringLibrary/sink_edge_checker_scope  mask{shortestPathTz=2*Tz_dif+2*Tz_pre+Tz_il}
      mask prompts: shortestPathTz "Sum of Tz on the path to the closest source"
      mask Display: disp(['pathTz = ', get_param(gcb,'shortestPathTz')])
  sinks6 : Subsystem  AncestorBlock=MeasuringLibrary/sink_edge_checker_scope  mask{shortestPathTz=2*Tz_dif+2*Tz_pre+Tz_ir}
      mask prompts: shortestPathTz "Sum of Tz on the path to the closest source"
      mask Display: disp(['pathTz = ', get_param(gcb,'shortestPathTz')])
  sources : Subsystem  AncestorBlock=MeasuringLibrary/source_edge_checker_scope
  sources1 : Subsystem  AncestorBlock=MeasuringLibrary/source_edge_checker_scope
  sources2 : Subsystem  AncestorBlock=MeasuringLibrary/source_edge_checker_scope
  sources3 : Subsystem  AncestorBlock=MeasuringLibrary/source_edge_checker_scope
  sources4 : Subsystem  AncestorBlock=MeasuringLibrary/source_edge_checker_scope
  sources5 : Subsystem  AncestorBlock=MeasuringLibrary/source_edge_checker_scope
  sources6 : Subsystem  AncestorBlock=MeasuringLibrary/source_edge_checker_scope
  sources7 : Subsystem  AncestorBlock=MeasuringLibrary/source_edge_checker_scope
  to Sink A : EdgesLibrary/SE1x1  Rk=Rk  slope=2000
  to Sink A1 : EdgesLibrary/SE1x1  Rk=Rk  slope=2000
  to Sink A2 : EdgesLibrary/SE1x1  Rk=Rk  slope=2000
  to Sink B : EdgesLibrary/SE1x1  Rk=Rk  slope=2000
  to Sink B1 : EdgesLibrary/SE1x1  Rk=Rk  slope=2000
  to Sink B2 : EdgesLibrary/SE1x1  Rk=Rk  slope=2000
  to Sink C : EdgesLibrary/SE1x1  Rk=Rk  slope=2000
  to Sink C1 : EdgesLibrary/SE1x1  Rk=Rk  slope=2000
  to Sink C2 : EdgesLibrary/SE1x1  Rk=Rk  slope=2000
  to Sink D : EdgesLibrary/SE1x1  Rk=Rk  slope=2000
  wires:
  Cout3/2 -> from Source B1/1
  Chart1/2(enableAri4) -> [LenAr], Subsystem2/7(Ari4)
  Brs3/2 -> from Source B2/1
  Subsystem1/5(Ali yk) -> deadtimes2/2(edge), Ali/2
  Bo1/4 -> BoY1/1
  Co1/3 -> CoX1/1
  AinSplit1/3 -> Ain1/2
  Ali/7 -> AinSplit1/3
  Ali/2 -> deadtimes2/1(x0z), Subsystem1/12(Ali x0)
  Bo1/6 -> Subsystem1/1(Bo x)
  Subsystem1/18(Bo yk) -> Bo1/1
  from Source A1/1 -> Ain1/1
  Ari/7 -> AinSplit1/5
  Cin1/4 -> CinY1/1
  Subsystem1/2(Cl yk) -> Cl1/2, deadtimes/2(edge)
  SE1x6/1 -> Cout1/1
  Cin1/3 -> CinX1/1
  Cout1/7 -> SE1x6/3
  Subsystem1/4(Ao yk) -> Ao1/1
  Aout1/2 -> to Sink A1/1
  Sink A1/2 -> to Sink A1/3
  Cout1/6 -> SE1x6/2
  Co1/4 -> CoY1/1
  Cl1/6 -> CinSplit1/4
  Source C1/1 -> from Source C1/1
  Brs1/7 -> from Source B1/3
  Subsystem1/1(Cs yk) -> deadtimes1/2(edge), Cs/2
  Cl1/7 -> CinSplit1/5
  AinSplit1/1 -> Ali/1
  Sink C1/1 -> to Sink C1/2
  Brs1/3 -> BrsX1/1
  Sink C1/2 -> to Sink C1/3
  Cs/4 -> CsY/1
  to Sink A1/2 -> Aout1/2
  Ari/4 -> AriY/1
  Cin1/6 -> from Source C1/2
  Cs/6 -> CinSplit1/2
  SE1x5/2 -> Ao1/2
  Ali/6 -> AinSplit1/2
  Ao1/3 -> AoX1/1
  Cl1/4 -> ClY/1
  from Source B1/1 -> Brs1/1
  Ain1/3 -> AinX1/1
  Chart2/3(enableCl7) -> [RenCl], Subsystem1/8(Cl7)
  Subsystem1/19(Brs yk) -> Brs1/2, deadtimes4/2(edge)
  Aout1/7 -> SE1x5/3
  Ain1/7 -> from Source A1/3
  Ain1/2 -> AinSplit1/1
  Subsystem1/7(Brs) -> Chart2/5(Brs)
  Subsystem1/11(Cs) -> Chart2/4(Cs)
  Subsystem1/13(Brs_Co) -> Chart2/10(Brs_Co)
  Bo1/2 -> to Sink B1/1
  Ali/4 -> AliY/1
  CinSplit1/2 -> Cl1/1
  Subsystem1/14(Cs_Bo) -> Chart2/9(Cs_Bo)
  Subsystem1/16(Ari_Co) -> Chart2/7(Ari_Co)
  Cs/2 -> deadtimes1/1(x0z), Subsystem1/14(Cs x0)
  Co1/6 -> Subsystem1/16(Co x)
  to Sink B1/2 -> Bo1/2
  Ali/3 -> AliX/1
  Chart2/6(enableBrs12) -> [RenBr], Subsystem1/5(Brs12)
  Cin1/7 -> from Source C1/3
  Ain1/4 -> AinY1/1
  Cs/3 -> CsX/1
  Ao1/6 -> Subsystem1/10(Ao x)
  Sink A/1 -> to Sink A/2
  Subsystem1/17(Ali_Bo) -> Chart2/6(Ali_Bo)
  Ao/3 -> AoX/1
  Kz_long/1 -> Kzs/1  "Kz_long"
  Ain/4 -> AinY/1
  Ain/3 -> AinX/1
  Bo/2 -> SE1x2/1
  Ain/6 -> from Source A/2
  Al/3 -> AlX/1
  Bl/4 -> BlY/1
  from Source A/1 -> Ain/1
  Source A/1 -> from Source A/1
  Aout/3 -> AoutX/1
  Aout/6 -> SE1x1/2
  Ain1/6 -> from Source A1/2
  Bl/3 -> BlX/1
  Cin/7 -> from Source C/3
  to Sink A/2 -> Aout/2
  Co1/2 -> SE1x6/1
  Aout/4 -> AoutY/1
  Aout/7 -> SE1x1/3
  Ain/2 -> AinSplit/1
  Bl/7 -> BinSplit1/3
  DinSplit/2 -> Dl/1
  Ao/5 -> Terminator2/1
  Aout1/6 -> SE1x5/2
  Cin/3 -> CinX/1
  Din/5 -> Terminator34/1
  Subsystem/9(Do yk) -> Do/1
  Dl/1 -> Terminator30/1
  Ars/6 -> AinSplit/4
  Aout1/4 -> AoutY1/1
  Al/6 -> AinSplit/2
  Ain/5 -> Terminator7/1
  Bo/4 -> BoY/1
  Co/6 -> Subsystem/27(Co x)
  Cout/4 -> CoutY/1
  Cl/1 -> Terminator22/1
  Brs/5 -> Terminator48/1
  Bout/7 -> SE1x2/3
  Co/4 -> CoY/1
  Co/5 -> Terminator20/1
  Crs/4 -> CrsY/1
  SE1x2/1 -> Bout/1
  CinSplit/3 -> Cin/2
  Cl/6 -> CinSplit/4
  Ao/4 -> AoY/1
  Bo1/3 -> BoX1/1
  Cout/5 -> Terminator23/1
  Bo1/7 -> Subsystem1/2(Bo Kz)
  Din/6 -> from Source D/2
  Bl/2 -> deadtimes9/1(x0z), Subsystem/3(Bl x0)
  Drs/1 -> Terminator31/1
  SE1x3/1 -> Cout/1
  Crs/6 -> CinSplit/2
  from Source C/1 -> Cin/1
  Cout/7 -> SE1x3/3
  Subsystem1/10(Cl) -> Chart2/3(Cl)
  Co1/7 -> Subsystem1/17(Co Kz)
  Cs/7 -> CinSplit1/3
  Ari/3 -> AriX/1
  Chart2/4(enableCs8) -> [RenCs], Subsystem1/9(Cs8)
  Cin1/2 -> CinSplit1/1
  SE1x5/1 -> Aout1/1
  Cin/6 -> from Source C/2
  Chart2/1(enableAli3) -> [RenAl], Subsystem1/6(Ali3)
  Tz_pre/1 -> Tzs/2  "Tz_pre"
  Cl1/3 -> ClX1/1
  Brs/3 -> BrsX/1
  Do/4 -> DoY/1
  to Sink D/2 -> Dout/2
  Ars/4 -> ArsY/1
  Din/4 -> DinY/1
  to Sink C/2 -> Cout/2
  to Sink D/1 -> sinks4/1(edge)
  Aout/2 -> to Sink A/1
  Cout1/3 -> CoutX1/1
  Ain/7 -> from Source A/3
  Drs/3 -> DrsX/1
  Dout/3 -> DoutX/1
  Subsystem/1(Crs yk) -> deadtimes8/2(edge), Crs/2
  Source D/1 -> from Source D/1
  Ars/7 -> AinSplit/5
  Brs1/4 -> BrsY1/1
  Dl/4 -> DlY/1
  Bin/3 -> BinX/1
  Dout/4 -> DoutY/1
  Dl/5 -> Terminator43/1
  DinSplit/1 -> Drs/1
  Bin/7 -> from Source B/3
  from Source D/2 -> sources5/1(edge)
  Dl/6 -> DinSplit/4
  Din/2 -> DinSplit/1
  Cl/7 -> CinSplit/5
  Sink D/2 -> to Sink D/3
  Ao/2 -> SE1x1/1
  Ari/2 -> Subsystem1/13(Ari x0), deadtimes3/1(x0z)
  Do/2 -> SE1x4/1
  SE1x2/2 -> Bo/2
  Din/1 -> Terminator28/1
  Ari1/4 -> AriY1/1
  Dl/3 -> DlX/1
  Co/1 -> Terminator39/1
  Bo/7 -> Subsystem/2(Bo Kz)
  Tz_long/1 -> Tzs/1  "Tz_long"
  Do/5 -> Terminator29/1
  Do/3 -> DoX/1
  Al/2 -> deadtimes5/1(x0z), Subsystem/23(Al x0)
  Kz_dif/1 -> Kzs/3  "Kz_dif"
  Brs/2 -> deadtimes10/1(x0z), Subsystem/4(Brs x0)
  BinSplit1/1 -> Bl/1
  Ars/3 -> ArsX/1
  Cin/1 -> Terminator19/1
  Sink A1/1 -> to Sink A1/2
  AinSplit/2 -> Ars/1
  Bout/1 -> Terminator15/1
  Cout1/4 -> CoutY1/1
  Brs1/2 -> deadtimes4/1(x0z), Subsystem1/3(Brs x0)
  Subsystem/5(Al yk) -> deadtimes5/2(edge), Al/2
  Co/3 -> CoX/1
  Crs/1 -> Terminator21/1
  SE1x1/1 -> Aout/1
  Crs/7 -> CinSplit/3
  Cout1/2 -> to Sink C1/1
  Crs/5 -> Terminator37/1
  Al/4 -> AlY/1
  Cout/3 -> CoutX/1
  Subsystem1/15(Cl_Ao) -> Chart2/8(Cl_Ao)
  Co/7 -> Subsystem/28(Co Kz)
  Bout/5 -> Terminator14/1
  Subsystem1/6(Ari yk) -> Ari/2, deadtimes3/2(edge)
  Bout/2 -> to Sink B/1
  from Source B/1 -> Bin/1
  Cl/4 -> Cly/1
  Dl/7 -> DinSplit/5
  Chart2/5(enableBrs11) -> [RenBs], Subsystem1/4(Brs11)
  Subsystem/2(Cl yk) -> deadtimes7/2(edge), Cl/2
  Dout/6 -> SE1x4/2
  Bin/6 -> from Source B/2
  Crs/2 -> deadtimes8/1(x0z), Subsystem/25(Crs x0)
  BinSplit1/2 -> Brs/1
  Bin/5 -> Terminator16/1
  from Source D/1 -> Din/1
  Ain/1 -> Terminator1/1
  Cl/3 -> ClX/1
  AinSplit/1 -> Al/1
  Cl/2 -> deadtimes7/1(x0z), Subsystem/26(Cl x0)
  Drs/2 -> deadtimes17/1(x0z), Subsystem/5(Drs x0)
  DinSplit/3 -> Din/2
  Ari/6 -> AinSplit1/4
  BinSplit1/3 -> Bin/2
  Do/6 -> Subsystem/7(Do x)
  Subsystem/3(Co yk) -> Co/1
  Bout/3 -> BoutX/1
  Do/7 -> Subsystem/8(Do Kz)
  Subsystem/7(Drs yk) -> deadtimes17/2(edge), Drs/2
  Brs/1 -> Terminator13/1
  Sink D/1 -> to Sink D/2
  Bl/5 -> Terminator47/1
  Cin/2 -> CinSplit/1
  Bo/6 -> Subsystem/1(Bo x)
  Subsystem/32(Brs yk) -> deadtimes10/2(edge), Brs/2
  Al/5 -> Terminator40/1
  Co/2 -> SE1x3/1
  Bo/1 -> Terminator46/1
  Din/7 -> from Source D/3
  Ars/5 -> Terminator41/1
  Bo/3 -> BoX/1
  Sink A/2 -> to Sink A/3
  Ao1/2 -> SE1x5/1
  Brs/4 -> BrsY/1
  Bin/2 -> BinSplit1/1
  Ao/1 -> Terminator42/1
  Al/7 -> AinSplit/3
  Dl/2 -> deadtimes16/1(x0z), Subsystem/6(Dl x0)
  Cs1/2 -> deadtimes15/1(x0z), Subsystem2/14(Cs x0)
  to Sink A/1 -> sinks3/1(edge)
  Bin/1 -> Terminator10/1
  Ao2/2 -> SE1x7/1
  to Sink C/1 -> Cout3/1
  Drs/6 -> DinSplit/2
  Cl/5 -> Terminator38/1
  from Source A/2 -> sources4/1(edge)
  Subsystem2/9(Ari) -> Chart1/2(Ari)
  Ao2/4 -> AoY2/1
  Ari1/3 -> AriX1/1
  Brs1/6 -> from Source B1/2
  Co2/7 -> Subsystem2/17(Co Kz)
  Subsystem2/10(Cl) -> Chart1/3(Cl)
  Subsystem/4(Ao yk) -> Ao/1
  Ali1/4 -> AliY1/1
  CinSplit2/2 -> Cl2/1
  Subsystem2/16(Ari_Co) -> Chart1/7(Ari_Co)
  CinSplit1/1 -> Cs/1
  Subsystem2/13(Brs_Co) -> Chart1/10(Brs_Co)
  Subsystem2/8(Ali) -> Chart1/1(Ali)
  Brs/6 -> BinSplit1/4
  Ain2/2 -> AinSplit2/1
  Subsystem2/11(Cs) -> Chart1/4(Cs)
  SE1x7/1 -> Aout2/1
  Cout2/3 -> CoutX2/1
  Aout2/7 -> SE1x7/3
  Drs/7 -> DinSplit/3
  Ain2/3 -> AinX2/1
  Chart1/3(enableCl7) -> [LenCl], Subsystem2/8(Cl7)
  Source A2/1 -> from Source A2/1
  Ao2/3 -> AoX2/1
  Do/1 -> Terminator45/1
  Cs1/6 -> CinSplit2/2
  Dout/7 -> SE1x4/3
  Ali1/6 -> AinSplit2/2
  Ao/6 -> Subsystem/21(Ao x)
  Aout/5 -> Terminator5/1
  Aout1/3 -> AoutX1/1
  to Sink A2/2 -> Aout2/2
  CinSplit/1 -> Crs/1
  Rk/1 -> Tzs1/1  "Rk"
  from Source B2/1 -> Brs2/1
  Brs2/3 -> BrsX2/1
  Brs2/4 -> BrsY2/1
  Brs2/2 -> Subsystem2/3(Brs x0), deadtimes11/1(x0z)
  Source A1/1 -> from Source A1/1
  Bo2/3 -> BoX2/1
  Cs1/7 -> CinSplit2/3
  Cout2/4 -> CoutY2/1
  Cs1/4 -> CsY1/1
  Ao1/4 -> AoY1/1
  Sink C2/2 -> to Sink C2/3
  Cout/2 -> to Sink C/1
  CinSplit2/3 -> Cin2/2
  Dout/2 -> to Sink D/1
  to Sink C1/2 -> Cout1/2
  AinSplit2/1 -> Ali1/1
  Subsystem/6(Ars yk) -> deadtimes6/2(edge), Ars/2
  Brs2/7 -> from Source B2/3
  SE1x6/2 -> Co1/2
  Cl2/7 -> CinSplit2/5
  Cl2/6 -> CinSplit2/4
  Bl/6 -> BinSplit1/2
  Subsystem1/3(Co yk) -> Co1/1
  Sink C2/1 -> to Sink C2/2
  Bin/4 -> BinY/1
  CinSplit2/1 -> Cs1/1
  Subsystem2/1(Cs yk) -> deadtimes15/2(edge), Cs1/2
  AinSplit2/2 -> Ari1/1
  Source C2/1 -> from Source C2/1
  Bo2/2 -> to Sink B2/1
  Cin/4 -> CinY/1
  Bout/4 -> BoutY/1
  Subsystem2/3(Co yk) -> Co2/1
  Bo2/7 -> Subsystem2/2(Bo Kz)
  Ao/7 -> Subsystem/22(Ao Kz)
  AinSplit/3 -> Ain/2
  Aout2/2 -> to Sink A2/1
  Co2/4 -> CoY2/1
  Subsystem2/14(Cs_Bo) -> Chart1/9(Cs_Bo)
  Drs/4 -> DrsY/1
  Subsystem2/4(Ao yk) -> Ao2/1
  Dout/1 -> Terminator33/1
  Sink A2/1(x) -> to Sink A2/2
  Cin/5 -> Terminator25/1
  Cout2/6 -> SE1x8/2
  Cout2/7 -> SE1x8/3
  SE1x8/2 -> Co2/2
  Cin2/3 -> CinX2/1
  Bout/6 -> SE1x2/2
  Subsystem2/2(Cl yk) -> deadtimes14/2(edge), Cl2/2
  Al/1 -> Terminator3/1
  Tz_dif/1 -> Tzs/3  "Tz_dif"
  SE1x8/1 -> Cout2/1
  Cin2/4 -> CinY2/1
  Ari1/7 -> AinSplit2/5
  SE1x7/2 -> Ao2/2
  CinSplit/2 -> Cl/1
  Ali1/7 -> AinSplit2/3
  Subsystem1/8(Ali) -> Chart2/1(Ali)
  from Source A2/1 -> Ain2/1
  AinSplit2/3 -> Ain2/2
  Ain2/6 -> from Source A2/2
  SE1x3/2 -> Co/2
  Drs/5 -> Terminator44/1
  from Source B1/2 -> Cout3/2
  Cout/1 -> Terminator24/1
  to Sink B2/1 -> Bo3/1
  Bo3/6 -> to Sink B2/2
  to Sink C2/2 -> Cout2/2
  Brs/7 -> BinSplit1/5
  Cin3/2 -> from Source C/1
  Brs3/6 -> to Sink B/2
  Brs3/7 -> to Sink B/3
  Ain2/7 -> from Source A2/3
  Cout3/6 -> to Sink C/2
  Subsystem/30(Bo yk) -> Bo/1
  Bo3/7 -> to Sink B2/3
  from Source C/2 -> Cin3/2
  Crs/3 -> CrsX/1
  Aout2/6 -> SE1x7/2
  Chart1/4(enableCs8) -> [LenCs], Subsystem2/9(Cs8)
  Co2/2 -> SE1x8/1
  Chart1/5(enableBrs11) -> [LenBs], Subsystem2/4(Brs11)
  Ars/2 -> Subsystem/24(Ars x), deadtimes6/1(x0z)
  Subsystem1/12(Brs_Ao) -> Chart2/11(Brs_Ao)
  Chart1/6(enableBrs12) -> [LenBr], Subsystem2/5(Brs12)
  to Sink B/1 -> Brs3/1
  Brs2/6 -> from Source B2/2
  Subsystem2/19(Brs yk) -> deadtimes11/2(edge), Brs2/2
  Subsystem2/15(Cl_Ao) -> Chart1/8(Cl_Ao)
  Sink A2/2(Kz) -> to Sink A2/3
  Ao2/6 -> Subsystem2/10(Ao x)
  Ari1/6 -> AinSplit2/4
  Bl/1 -> Terminator12/1
  Cin2/7 -> from Source C2/3
  from Source B2/2 -> Brs3/2
  Dout/5 -> Terminator32/1
  Ain2/4 -> AinY2/1
  Bo2/4 -> BoY2/1
  Cin2/6 -> from Source C2/2
  from Source C2/1 -> Cin2/1
  Chart1/1(enableAli3) -> [LenAl], Subsystem2/6(Ali3)
  to Sink B2/2 -> Bo2/2
  Subsystem2/12(Brs_Ao) -> Chart1/11(Brs_Ao)
  Cin3/7 -> to Sink B1/3
  SE1x4/1 -> Dout/1
  Cs1/3 -> CsX1/1
  Cout/6 -> SE1x3/2
  Ali1/2 -> deadtimes12/1(x0z), Subsystem2/12(Ali x0)
  Cl2/2 -> Subsystem2/15(Cl x0), deadtimes14/1(x0z)
  Ao2/7 -> Subsystem2/11(Ao Kz)
  Subsystem2/18(Bo yk) -> Bo2/1
  Cl2/4 -> ClY1/1
  Aout2/3 -> AoutX2/1
  from Source C1/1 -> Cin1/1
  Ari1/2 -> Subsystem2/13(Ari x0), deadtimes13/1(x0z)
  Bo/5 -> Terminator11/1
  Subsystem2/17(Ali_Bo) -> Chart1/6(Ali_Bo)
  SE1x1/2 -> Ao/2
  Co2/3 -> CoX2/1
  Ao1/7 -> Subsystem1/11(Ao Kz)
  Cin2/2 -> CinSplit2/1
  Subsystem1/9(Ari) -> Chart2/2(Ari)
  Bo2/6 -> Subsystem2/1(Bo x)
  Aout/1 -> Terminator6/1
  Ali1/3 -> AliX1/1
  Cout2/2 -> to Sink C2/1
  Din/3 -> DinX/1
  Cout3/7 -> to Sink C/3
  Subsystem2/7(Brs) -> Chart1/5(Brs)
  Ars/1 -> Terminator4/1
  Aout2/4 -> AoutY2/1
  from Source B/2 -> Bo3/2
  Cl1/2 -> deadtimes/1(x0z), Subsystem1/15(Cl x0)
  Subsystem2/5(Ali yk) -> Ali1/2, deadtimes12/2(edge)
  Subsystem/8(Dl yk) -> deadtimes16/2(edge), Dl/2
  to Sink B/2 -> Bout/2
  Subsystem2/6(Ari yk) -> deadtimes13/2(edge), Ari1/2
  Bo3/2 -> from Source B/1
  Kz_pre/1 -> Kzs/2  "Kz_pre"
  SE1x4/2 -> Do/2
  Cin3/6 -> to Sink B1/2
  Co2/6 -> Subsystem2/16(Co x)
  CinSplit1/3 -> Cin1/2
  Cl2/3 -> ClX2/1
  to Sink B1/1 -> Cin3/1
  AinSplit1/2 -> Ari/1
  Subsystem/10(Al) -> Plus-Controller/3(Al)
  Subsystem/11(Ars) -> Plus-Controller/4(Ars)
  Subsystem/12(Bl) -> Plus-Controller/1(Bl)
  Subsystem/13(Brs) -> Plus-Controller/2(Brs)
  Subsystem/14(Cl) -> Plus-Controller/5(Cl)
  Subsystem/15(Crs) -> Plus-Controller/6(Crs)
  Subsystem/16(Dl) -> Plus-Controller/7(Dl)
  Subsystem/17(Drs) -> Plus-Controller/8(Drs)
  Subsystem/18(Al_Bo) -> Plus-Controller/9(Al_Bo)
  Subsystem/19(Ars_Do) -> Plus-Controller/10(Ars_Do)
  Subsystem/20(Ars_Co) -> Plus-Controller/11(Ars_Co)
  Subsystem/21(Bl_Do) -> Plus-Controller/12(Bl_Do)
  Subsystem/22(Brs_Co) -> Plus-Controller/13(Brs_Co)
  Subsystem/23(Brs_Ao) -> Plus-Controller/14(Brs_Ao)
  Subsystem/24(Cl_Ao) -> Plus-Controller/15(Cl_Ao)
  Subsystem/25(Crs_Bo) -> Plus-Controller/16(Crs_Bo)
  Subsystem/26(Crs_Do) -> Plus-Controller/17(Crs_Do)
  Subsystem/27(Dl_Co) -> Plus-Controller/18(Dl_Co)
  Subsystem/28(Drs_Ao) -> Plus-Controller/19(Drs_Ao)
  Subsystem/29(Drs_Bo) -> Plus-Controller/20(Drs_Bo)
  Plus-Controller/1(enAl) -> [CenAl], Subsystem/9(enAl)
  Plus-Controller/2(enAs) -> [CenAs], Subsystem/10(enAs)
  Plus-Controller/3(enAr) -> [CenAr], Subsystem/11(enAr)
  Plus-Controller/5(enBs) -> [CenBs], Subsystem/13(enBs)
  Plus-Controller/6(enBr) -> [CenBr], Subsystem/14(enBr)
  Plus-Controller/7(enCl) -> [CenCl], Subsystem/15(enCl)
  Plus-Controller/8(enCs) -> [CenCs], Subsystem/16(enCs)
  Plus-Controller/9(enCr) -> [CenCr], Subsystem/17(enCr)
  Plus-Controller/10(enDl) -> [CenDl], Subsystem/18(enDl)
  Plus-Controller/11(enDs) -> Subsystem/19(enDs), [CenDs]
  Plus-Controller/12(enDr) -> [CenDr], Subsystem/20(enDr)
  from Source C1/2 -> sources1/1(edge)
  from Source A1/2 -> sources2/1(edge)
  from Source A2/2 -> sources6/1(edge)
  from Source C2/2 -> sources7/1(edge)
  to Sink C1/1 -> sinks1/1(edge)
  to Sink A1/1 -> sinks2/1(edge)
  to Sink A2/1 -> sinks5/1(edge)
  to Sink C2/1 -> sinks6/1(edge)
  Plus-Controller/4(enBl) -> [CenBl], Subsystem/12(enBl)
  Chart2/2(enableAri4) -> [RenAr], Subsystem1/7(Ari4)
  [RenCs] -> deadtimes1/3(edge_enablestate)
  [RenCl] -> deadtimes/3(edge_enablestate)
  [RenAl] -> deadtimes2/3(edge_enablestate)
  [RenAr] -> deadtimes3/3(edge_enablestate)
  [RenBr] -> Logical Operator/1
  [RenBs] -> Logical Operator/2
  Logical Operator/1 -> deadtimes4/3(edge_enablestate)
  [LenCs] -> deadtimes15/3(edge_enablestate)
  [LenCl] -> deadtimes14/3(edge_enablestate)
  [LenBs] -> Logical Operator1/1
  [LenBr] -> Logical Operator1/2
  Logical Operator1/1 -> deadtimes11/3(edge_enablestate)
  [LenAr] -> deadtimes13/3(edge_enablestate)
  [LenAl] -> deadtimes12/3(edge_enablestate)
  [CenCl] -> deadtimes7/3(edge_enablestate)
  [CenCr] -> Logical Operator2/2
  [CenCs] -> Logical Operator2/1
  Logical Operator2/1 -> deadtimes8/3(edge_enablestate)
  [CenAl] -> deadtimes5/3(edge_enablestate)
  Logical Operator3/1 -> deadtimes6/3(edge_enablestate)
  [CenAs] -> Logical Operator3/1
  [CenAr] -> Logical Operator3/2
  [CenBs] -> Logical Operator4/1
  [CenBr] -> Logical Operator4/2
  Subsystem/31(Bl yk) -> deadtimes9/2(edge), Bl/2
  [CenBl] -> deadtimes9/3(edge_enablestate)
  Logical Operator4/1 -> deadtimes10/3(edge_enablestate)
  [CenDl] -> deadtimes16/3(edge_enablestate)
  [CenDs] -> Logical Operator5/1
  [CenDr] -> Logical Operator5/2
  Logical Operator5/1 -> deadtimes17/3(edge_enablestate)
  [CenAl] -> Scope/1
  [CenAs] -> Scope/2
  [CenAr] -> Scope/3
  [CenBl] -> Scope/4
  [CenBs] -> Scope/5
  [CenBr] -> Scope/6
  [CenCl] -> Scope/7
  [CenCs] -> Scope/8
  [CenCr] -> Scope/9
  [CenDl] -> Scope/10
  [CenDs] -> Scope/11
  [CenDr] -> Scope/12

== system Scenario_MinimumExample_TwithoutTrafficLights_tol/Sink A2 ==
  Constant : Constant  Value=0
  Constant1 : Constant
  x : Outport
  Kz : Outport  Port=2
  wires:
  Constant1/1 -> Kz/1
  Constant/1 -> x/1
